simulink model "n_trotinettes_crash"  (Simulink 6.5)
settings: Solver=ode45  StartTime=0.0  StopTime=L  RelTol=1e-6
undefined symbols (not defined in the file or in its folder): Delta, Ig, K, Ka, Ki, Ktach, Kv, L, M_ecart, N
settings Model: Creator=admin  LastModifiedBy=admin
settings DataIOCC: SignalLoggingName=sigsOut
settings DebuggingCC: SolverPrmCheckMsg=none  MultiTaskDSMMsg=warning  MultiTaskCondExecSysMsg=none  StrictBusMsg=None
settings HardwareCC: TargetUnknown=on
settings RTWCC: IncludeERTFirstTime=on

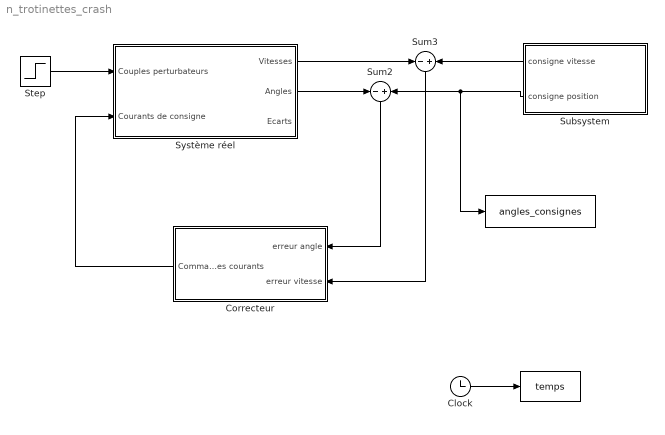
== system n_trotinettes_crash ==
  " " : ToWorkspace  VariableName=temps  SampleTime=-1  SaveFormat=Array
  "  " : ToWorkspace  VariableName=angles_consignes  SampleTime=-1  SaveFormat=Array
  Clock : Clock
      settings: Decimation=10
  Correcteur : Subsystem  Orientation=left
  Step : Step  Time=L*0.1  Before=zeros(N,1)  After=ones(N,1)  SampleTime=0
  Subsystem : Subsystem  Orientation=left
  Sum2 : Sum  Orientation=down  Inputs=-|+  SaturateOnIntegerOverflow=on
  Sum3 : Sum  Orientation=down  Inputs=-|+  SaturateOnIntegerOverflow=on
  Système réel : Subsystem
  wires:
  Step/1 -> Système réel/1(Couples perturbateurs)
  Système réel/2(Angles) -> Sum2/1
  Subsystem/2(consigne position) -> Sum2/2, "  "/1
  Clock/1 -> " "/1
  Correcteur/1(Commandes courants) -> Système réel/2(Courants de consigne)
  Système réel/1(Vitesses) -> Sum3/1
  Sum3/1 -> Correcteur/2(erreur vitesse)
  Sum2/1 -> Correcteur/1(erreur angle)
  Subsystem/1(consigne vitesse) -> Sum3/2

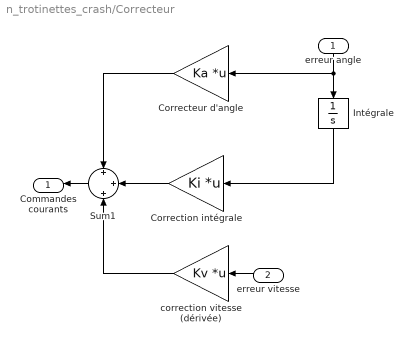
== system n_trotinettes_crash/Correcteur ==
  erreur angle : Inport  Orientation=down
  erreur vitesse : Inport  Orientation=left  Port=2
  Correcteur d'angle : Gain  Orientation=left  Gain=Ka  Multiplication=Matrix(K*u)  SaturateOnIntegerOverflow=on
  Correction intégrale : Gain  Orientation=left  Gain=Ki  Multiplication=Matrix(K*u)  SaturateOnIntegerOverflow=on
  Intégrale : Integrator  Orientation=down  InitialCondition=zeros(N,1)
  Sum1 : Sum  Orientation=left  Inputs=+|+|+  SaturateOnIntegerOverflow=on
  correction vitesse (dérivée) : Gain  Orientation=left  Gain=Kv  Multiplication=Matrix(K*u)  SaturateOnIntegerOverflow=on
  Commandes courants : Outport  Orientation=left
  wires:
  erreur angle/1 -> Correcteur d'angle/1, Intégrale/1
  Correcteur d'angle/1 -> Sum1/1
  Intégrale/1 -> Correction intégrale/1
  correction vitesse (dérivée)/1 -> Sum1/3
  Correction intégrale/1 -> Sum1/2
  Sum1/1 -> Commandes courants/1
  erreur vitesse/1 -> correction vitesse (dérivée)/1

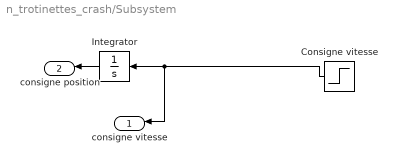
== system n_trotinettes_crash/Subsystem ==
  Consigne vitesse : Step  Orientation=left  Time=L/2  Before=zeros(N,1)  After=ones(N,1)  SampleTime=0
  Integrator : Integrator  Orientation=left  InitialCondition=[0:N-1]'*Delta
  consigne vitesse : Outport  Orientation=left
  consigne position : Outport  Orientation=left  Port=2
  wires:
  Consigne vitesse/1 -> Integrator/1, consigne vitesse/1
  Integrator/1 -> consigne position/1

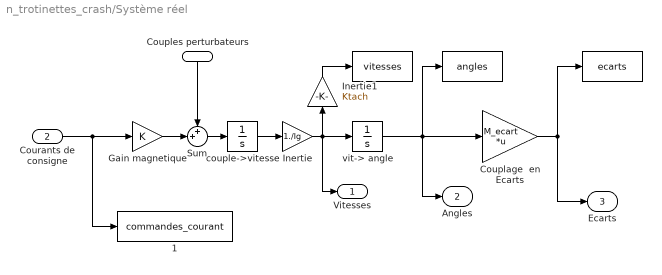
== system n_trotinettes_crash/Système réel ==
  Couples perturbateurs : Inport  Orientation=down
  Courants de consigne : Inport  Port=2
  " " : ToWorkspace  VariableName=vitesses  SampleTime=-1  SaveFormat=Array
  "  " : ToWorkspace  VariableName=angles  SampleTime=-1  SaveFormat=Array
  "   " : ToWorkspace  VariableName=ecarts  SampleTime=-1  SaveFormat=Array
  "   1" : ToWorkspace  VariableName=commandes_courant  SampleTime=-1  SaveFormat=Array
  Couplage  en Ecarts : Gain  Gain=M_ecart  Multiplication=Matrix(K*u)  SaturateOnIntegerOverflow=on
  Gain magnetique : Gain  Gain=K  SaturateOnIntegerOverflow=on
  Inertie : Gain  Gain=1./Ig  SaturateOnIntegerOverflow=on
  Inertie1 : Gain  Orientation=up  Gain=Ktach  SaturateOnIntegerOverflow=on
  Sum : Sum  Inputs=++|  SaturateOnIntegerOverflow=on
  couple->vitesse : Integrator  InitialCondition=zeros(N,1)
  vit-> angle : Integrator  InitialCondition=(0:N-1)*Delta
  Vitesses : Outport
  Angles : Outport  Port=2
  Ecarts : Outport  Port=3
  wires:
  couple->vitesse/1 -> Inertie/1
  Gain magnetique/1 -> Sum/2
  Sum/1 -> couple->vitesse/1
  vit-> angle/1 -> "  "/1, Angles/1, Couplage  en Ecarts/1
  Couples perturbateurs/1 -> Sum/1
  Courants de consigne/1 -> Gain magnetique/1, "   1"/1
  Couplage  en Ecarts/1 -> "   "/1, Ecarts/1
  Inertie/1 -> vit-> angle/1, Vitesses/1, Inertie1/1
  Inertie1/1 -> " "/1
